simulink model "omni_3DOF_PD"  (R2023a)
settings: Solver=VariableStepAuto  StartTime=0.0  StopTime=40  RelTol=1e-3
libraries: robotcorelib x1
settings Model: Creator=Adan Daniel  LastModifiedBy=Adan Daniel

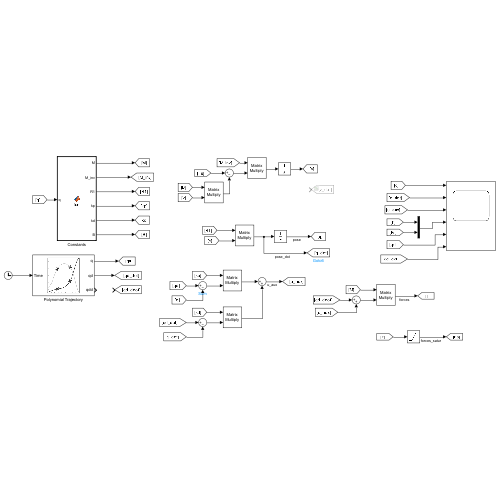
[thumbnail: Simulink's stored preview of the top-level diagram]
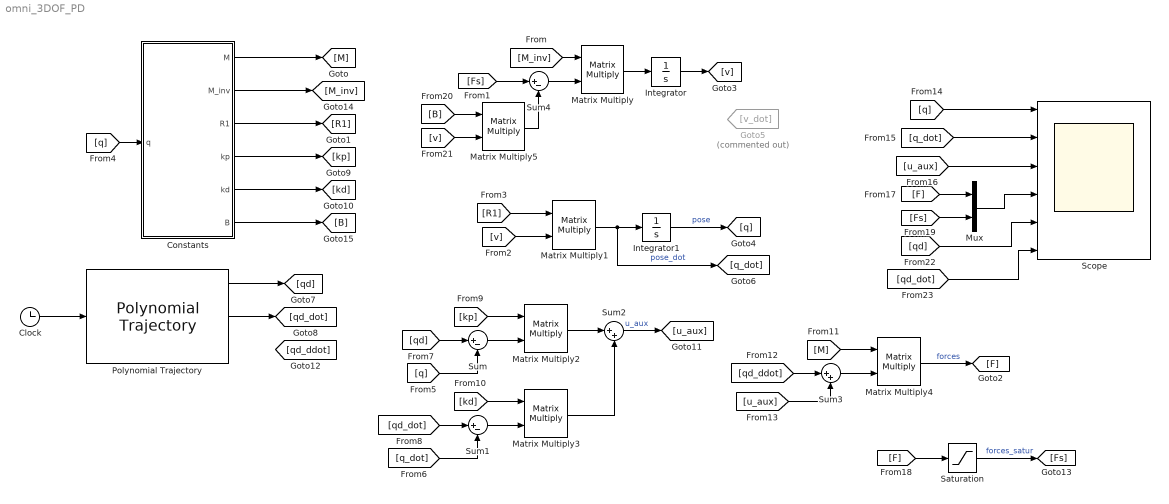
== system omni_3DOF_PD ==
  Clock : Clock
  Constants : MATLAB Function  TreatAsAtomicUnit=on
  Goto5 : Goto  Commented=on  GotoTag=v_dot
  Integrator : Integrator  InitialCondition=[0; 0; 0]
  Integrator1 : Integrator  InitialCondition=[0; 0; 0]
  Matrix Multiply{,1..5} (6 alike) : Product  Multiplication=Matrix(*)
  Mux : Mux  Inputs=2
  Polynomial Trajectory : robotcorelib/Polynomial Trajectory  WaypointSource=Internal  Waypoints=[2, 2, 2; 0, 2, 2; 0, 0, 0]  TimePoints=[10, 20, 30]  TimeInterval=[ 1, 4 ]  Method=Cubic Polynomial  ParameterSource=Internal  VelocityBoundaryCondition=zeros( 3, 3 )  AccelerationBoundaryCondition=zeros( 2, 5 )  SimulateUsing=Interpreted execution
  Saturation : Saturate  UpperLimit=[1; 1; 0.5]  LowerLimit=[-1; -1; -0.5]
  Scope : Scope  NumInputPorts=6
  Sum : Sum  Inputs=|+-
  Sum1 : Sum  Inputs=|+-
  Sum2 : Sum  Inputs=|++
  Sum3 : Sum  Inputs=|++
  Sum4 : Sum  Inputs=|+-
  wires:
  Constants/1(M) -> [M]
  Constants/3(R1) -> [R1]
  Integrator/1 -> [v]
  [R1] -> Matrix Multiply1/1
  Integrator1/1 -> [q]  "pose"
  [v] -> Matrix Multiply1/2
  [q] -> Constants/1(q)
  Matrix Multiply1/1 -> [q_dot], Integrator1/1  "pose_dot"
  [qd] -> Sum/1
  [q] -> Sum/2
  [q_dot] -> Sum1/2
  [qd_dot] -> Sum1/1
  Constants/4(kp) -> [kp]
  Constants/5(kd) -> [kd]
  Sum1/1 -> Matrix Multiply3/2
  [kd] -> Matrix Multiply3/1
  [kp] -> Matrix Multiply2/1
  Sum/1 -> Matrix Multiply2/2
  Matrix Multiply2/1 -> Sum2/1
  Matrix Multiply3/1 -> Sum2/2
  Sum2/1 -> [u_aux]  "u_aux"
  [qd_ddot] -> Sum3/1
  [u_aux] -> Sum3/2
  Matrix Multiply4/1 -> [F]  "forces"
  [M] -> Matrix Multiply4/1
  Sum3/1 -> Matrix Multiply4/2
  [q] -> Scope/1
  [q_dot] -> Scope/2
  [u_aux] -> Scope/3
  [F] -> Saturation/1
  Saturation/1 -> [Fs]  "forces_satur"
  [F] -> Mux/1
  [Fs] -> Mux/2
  Mux/1 -> Scope/4
  Constants/2(M_inv) -> [M_inv]
  Clock/1 -> Polynomial Trajectory/1
  Polynomial Trajectory/1 -> [qd]
  Constants/6(B) -> [B]
  Polynomial Trajectory/2 -> [qd_dot]
  [v] -> Matrix Multiply5/2
  [B] -> Matrix Multiply5/1
  Matrix Multiply5/1 -> Sum4/2
  [Fs] -> Sum4/1
  Sum4/1 -> Matrix Multiply/2
  [M_inv] -> Matrix Multiply/1
  Matrix Multiply/1 -> Integrator/1
  [qd] -> Scope/5
  [qd_dot] -> Scope/6

== matlab function omni_3DOF_PD/Constants ==
  data: q input; M output; M_inv output; R1 output; kp output; kd output; B output
function [M, M_inv, R1, kp, kd, B] = fcn(q)


yaw = q(3);

m = 35; % kg
J = 1.39; % Kg * m^2

M = [m, 0, 0;
     0, m, 0;
     0, 0, J];

M_inv = inv(M);

R1 = [cos(yaw), -sin(yaw), 0;
      sin(yaw), cos(yaw), 0;
      0, 0, 1];

kp = [0.2, 0, 0;
     0, 0.2, 0;
     0, 0, 1];

kd = [1, 0, 0;
     0, 1, 0;
     0, 0, 1];

B = [3.73, 0, 0;
     0, 3.34, 0;
     0, 0, 0.73];
